simulink model "ALBERT01"  (R2024b)
settings: Solver=VariableStepAuto  StartTime=0.0  StopTime=10  RelTol=1e-3
libraries: simulink_extras x2, shared6dof x1
settings Model: Creator=felixzauner  LastModifiedBy=felixzauner

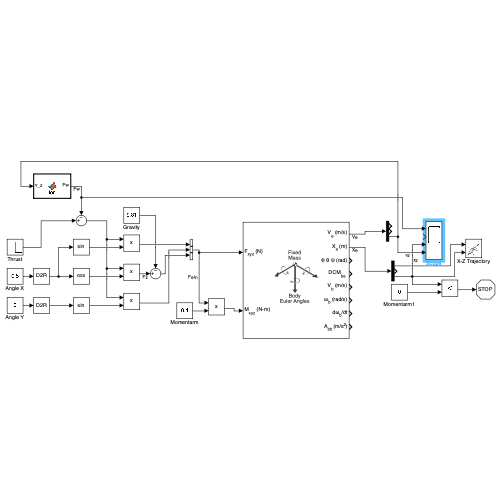
[thumbnail: Simulink's stored preview of the top-level diagram]
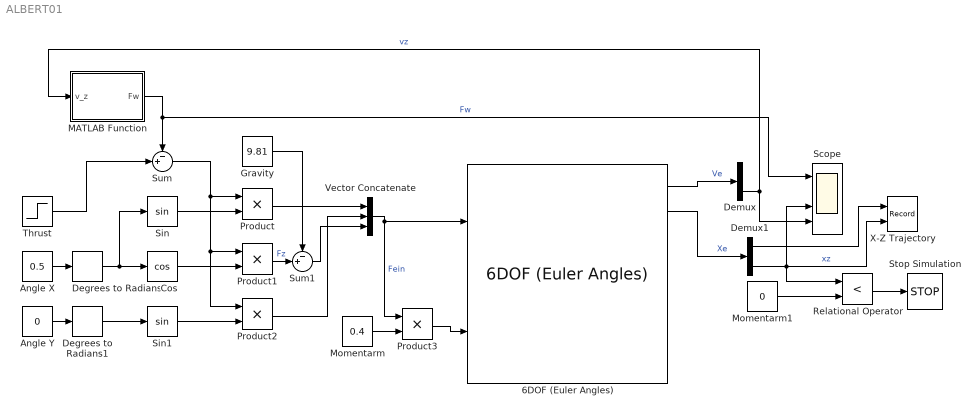
== system ALBERT01 ==
  6DOF (Euler Angles) : shared6dof/6DOF (Euler Angles)  units=Metric (MKS)  mtype=Fixed  rep=Euler Angles  xme_0=[0 0 0]  Vm_0=[0 0 0]  eul_0=[0 0 0]  pm_0=[0 0 0]  mass_0=1  mass_e=0.5  mass_f=2.0  inertia=eye(3)  inertia_e=eye(3)  inertia_f=2*eye(3)  k_quat=1.0  vre_flag=on  abi_flag=off  aMode=0  xme_statename=''  Vm_statename=''  eul_statename=''  quat_statename=''  pm_statename=''  mass_statename=''
  Angle X : Constant  Value=0.5
  Angle Y : Constant  Value=0
  Cos : Trigonometry  Operator=cos
  Degrees to Radians : simulink_extras/Transformations/Degrees to Radians
  Degrees to Radians1 : simulink_extras/Transformations/Degrees to Radians
  Demux : Demux  Outputs=3
  Demux1 : Demux  Outputs=3
  Gravity : Constant  Value=9.81
  MATLAB Function : MATLAB Function  TreatAsAtomicUnit=on
  Momentarm : Constant  Value=0.4
  Momentarm1 : Constant  Value=0
  Product{,1..3} (4 alike) : Product
  Relational Operator : RelationalOperator  Operator=<  OutDataTypeStr=boolean  RndMeth=Simplest  InputSameDT=off
  Scope : Scope  NumInputPorts=4
  Sin : Trigonometry
  Sin1 : Trigonometry
  Stop Simulation : Stop
  Sum : Sum  Inputs=-+|
  Sum1 : Sum  Inputs=-+|
  Thrust : Step  Time=2  Before=40  After=0  SampleTime=0
  Vector Concatenate : Concatenate  NumInputs=3
  X-Z Trajectory : Record  FileSettingsInternal="{\"entries\":[{\"content\":{\"excelSettings\":{\"content\":{},\"type\":\"Streamout.ExcelSettings\"}},\"type\":\"Streamout.FileSettingStorage\",\"uuid\":\"\"}],\"packageUris\":[\"http:\\/\\/schema.mathworks.com\\/mf0\\/streamout_blocks\\/R2020a\"],\"version\":\"1.0\"}"  Layout=[1 1]  SignalsInternal="{\"entries\":[{\"content\":{\"signals\":[{\"content\":{\"blockPath\":[],\"dimensions\":[1],\"domain\":\"\",\"lineColor\":\"#a2142f\",\"plots\":[ 1 ],\"port\":1,\"sid\":[\"\"],\"signalID\":1,\"signalName\":\"Demux1:1\"},\"type\":\"RecordBlkView.Signal\",\"uuid\":\"\"},{\"content\":{\"blockPath\":[],\"dimensions\":[1],\"domain\":\"\",\"lineColor\":\"#139fff\",\"plots\":[ 1 ],\"port\":2,\"sid\":[\"\"],\"signalID\":2,\"signalName\":\"xz\"},\"type\":\"RecordBlkView.Signal\",\"uuid\":\"\"}]},\"type\":\"RecordBlkView.InputSignals\",\"uuid\":\"\"}],\"packageUris\":[\"http:\\/\\/schema.mathworks.com\\/mf0\\/streamout_blocks\\/R2020a\"],\"version\":\"1.0\"}"  VisualizationBindings="{\"xyplotplugin\":{\"info\":[{\"series\":[{\"bindingParametersList\":[{\"parameter\":\"X-Axis\",\"signalID\":1,\"signalName\":\"Demux1:1\"},{\"parameter\":\"Y-Axis\",\"signalID\":2,\"signalName\":\"xz\"}],\"seriesID\":0}],\"subplotID\":1}]}}"  CompatibilityTag=XY  st=-1
  wires:
  Angle X/1 -> Degrees to Radians/1
  Degrees to Radians/1 -> Sin/1, Cos/1
  Cos/1 -> Product1/2
  Sin/1 -> Product/2
  Angle Y/1 -> Degrees to Radians1/1
  Degrees to Radians1/1 -> Sin1/1
  Sin1/1 -> Product2/2
  Product/1 -> Vector Concatenate/1
  Product2/1 -> Vector Concatenate/2
  Vector Concatenate/1 -> Product3/1, 6DOF (Euler Angles)/1  "Fein"
  Product3/1 -> 6DOF (Euler Angles)/2
  Momentarm/1 -> Product3/2
  6DOF (Euler Angles)/1 -> Demux/1  "Ve"
  Demux/3 -> MATLAB Function/1(v_z), Scope/4  "vz"
  Thrust/1 -> Sum/2
  Sum/1 -> Product2/1, Product1/1, Product/1
  MATLAB Function/1(Fw) -> Scope/1, Sum/1  "Fw"
  6DOF (Euler Angles)/2 -> Demux1/1  "Xe"
  Demux1/3 -> X-Z Trajectory/2, Scope/3, Relational Operator/1  "xz"
  Momentarm1/1 -> Relational Operator/2
  Relational Operator/1 -> Stop Simulation/1
  Product1/1 -> Sum1/2  "Fz"
  Sum1/1 -> Vector Concatenate/3
  Gravity/1 -> Sum1/1
  Demux1/1 -> X-Z Trajectory/1

== matlab function ALBERT01/MATLAB Function ==
  data: v_z input; Fw output
function Fw = fcn(v_z)

Fw = 0.5 * v_z^2 * 0.5 * 0.08^2 * 3.14
